simulink model "Galvo_CC_linmod_v30"  (R2013a)
settings: Solver=ode45  StartTime=0.0  StopTime=10.0  MaxStep=1e-4  RelTol=1e-3
settings Model: Creator=mainster  LastModifiedBy=mainster

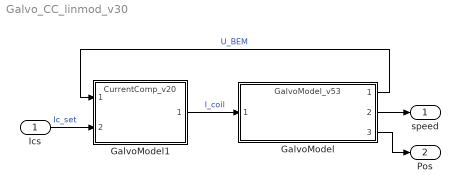
== system Galvo_CC_linmod_v30 ==
  Ics : Inport
  GalvoModel : ModelReference  ModelNameDialog=GalvoModel_v53.slx  Variant=on  OverrideUsingVariant=v53_neuer_cc  ModelReferenceVersion=1.59  CopyOfModelName=GalvoModel_v53.slx  DefaultDataLogging=on
      mask Display:
      | str=sprintf('%s',get(gcbh,'ModelName'));
      | port_label('input', 1, 'I_{Coil}','texmode','on')
      | color('blue');
      | port_label('output', 3, 'Pos','texmode','on')
      | color('black');
      | port_label('output', 2, 'Speed','texmode','on')
      | port_label('output', 1, 'U_{BEM}','texmode','on')
      | %text(.05,.98,['{\fontsize{12}\it\bf' strrep(str,'_',' ') '}'],'horizontalAlignment','left','verticalAlignment','top','texmode','on')
      | text(.015,.98,['{\fontsize{12}\it\bf' strrep(str,'_','\_') '}'],'horizontalAlignment','left','verticalAlignment','top','texmode','on')
      | text(.15,.05,['{\fontsize{10}\itmechanics}'],'horizontalAlignment','left','verticalAlignment','bottom','texmode','on')
  GalvoModel1 : ModelReference  ModelNameDialog=CurrentComp_v20.slx  Variant=on  OverrideUsingVariant=cc_v20  ModelReferenceVersion=1.73  CopyOfModelName=CurrentComp_v20.slx  DefaultDataLogging=on
      mask Display:
      | str=sprintf('%s',get(gcbh,'ModelName'));
      | port_label('input', 2, 'I_{Set Coil}','texmode','on')
      | color('red');
      | port_label('input', 1, 'U_{BEM}','texmode','on')
      | color('black');
      | port_label('output', 1, 'I_{Coil}','texmode','on')
      | %text(.05,.98,['{\fontsize{12}\it\bf' strrep(str,'_',' ') '}'],'horizontalAlignment','left','verticalAlignment','top','texmode','on')
      | text(.95,0.95,['{\fontsize{12}\it\bfG_{cc}(s)}'],'horizontalAlignment','right','verticalAlignment','top','texmode','on')
      | %text(.15,.05,['{\fontsize{10}\itmechanics}'],'horizontalAlignment','left','verticalAlignment','bottom','texmode','on')
  speed : Outport
  Pos : Outport  Port=2
  wires:
  GalvoModel/1 -> GalvoModel1/1  "U_BEM"
  Ics/1 -> GalvoModel1/2  "Ic_set"
  GalvoModel1/1 -> GalvoModel/1  "I_coil"
  GalvoModel/2 -> speed/1
  GalvoModel/3 -> Pos/1
